simulink model "Integrated_LKS"  (Simulink 10.2)
settings: Solver=ode4  StartTime=0.0  StopTime=30  FixedStep=0.005  RelTol=1e-3  EnableMultiTasking=on
undefined symbols (not defined in the file or in its folder): sigbuilder_block
libraries: simulink x2
settings Model: Creator=Infineon02  LastModifiedBy=user
settings DataIOCC: SignalLoggingName=sigsOut
settings OptimizationCC: ExpressionDepthLimit=2147483647  InitFltsAndDblsToZero=on
settings DebuggingCC: SaveWithParameterizedLinksMsg=none  SignalResolutionControl=TryResolveAllWithWarning  MultiTaskDSMMsg=warning  MultiTaskCondExecSysMsg=none  StateNameClashWarn=warning
settings HardwareCC: TargetUnknown=on
settings GRTTargetCC: TargetFcnLib=ansi_tfl_tmw.mat

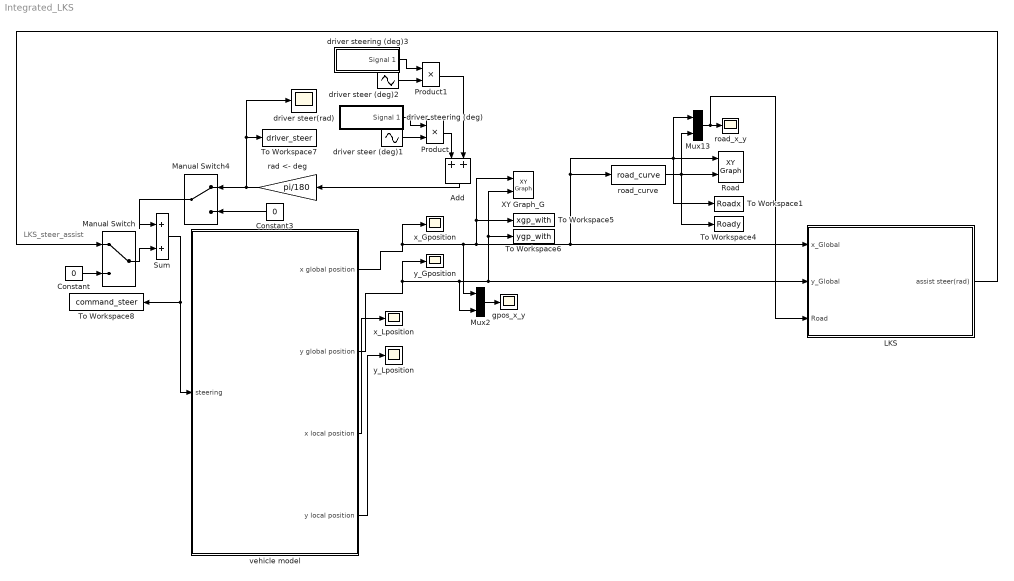
== system Integrated_LKS ==
  note: LKS_steer_assist
  Add : Sum
  Constant : Constant  Value=0
  Constant3 : Constant  Value=0
  LKS : Subsystem
  Manual Switch : ManualSwitch
  Manual Switch4 : ManualSwitch
  Mux13 : Mux  Inputs=2
  Mux2 : Mux  Inputs=2
  Product : Product  RndMeth=Zero
  Product1 : Product  RndMeth=Zero
  Road : simulink/Sinks/XY Graph  xmin=0  xmax=500  ymin=-100  ymax=1  st=0
  Sum : Sum  Inputs=|++  SaturateOnIntegerOverflow=on
  To Workspace1 : ToWorkspace  VariableName=Roadx  SampleTime=-1
  To Workspace4 : ToWorkspace  VariableName=Roady  SampleTime=-1
  To Workspace5 : ToWorkspace  VariableName=xgp_with  SampleTime=-1
  To Workspace6 : ToWorkspace  VariableName=ygp_with  SampleTime=-1
  To Workspace7 : ToWorkspace  VariableName=driver_steer  SampleTime=-1
  To Workspace8 : ToWorkspace  VariableName=command_steer  SampleTime=-1
  XY Graph_G : simulink/Sinks/XY Graph  xmin=0  xmax=500  ymin=-100  ymax=1  st=0
  driver steer (deg)1 : Sin  Amplitude=0.8  Frequency=0.34907  Phase=0.34898  SampleTime=0
  driver steer (deg)2 : Sin  Amplitude=0.8  Frequency=0.165347  Phase=2.64  SampleTime=0
  driver steer(rad) : Scope
  driver steering (deg) : Subsystem  Tag=STV Subsys  LoadFcn=sigbuilder_block('load');  StartFcn=sigbuilder_block('start');  StopFcn=sigbuilder_block('stop');  ClipboardFcn=sigbuilder_block('clipboard');  mask(Sigbuilder block){tuvar=[0:10]}
      mask help: Sigbuilder GUI
      mask init:
      | if ~strcmp(get_param(bdroot(gcbh),'SimulationStatus'),'stopped') tuvar = sigbuilder_block('maskInit'); end
      settings: CopyFcn=sigbuilder_block('copy');  DeleteFcn=sigbuilder_block('delete');  ModelCloseFcn=sigbuilder_block('modelClose');  PreSaveFcn=sigbuilder_block('preSave');  PauseFcn=sigbuilder_block('pause')  ContinueFcn=sigbuilder_block('continue')  NameChangeFcn=sigbuilder_block('namechange');  OpenFcn=sigbuilder_block('open',[-717 159.75 558.75 274.5 ]);  CloseFcn=sigbuilder_block('close');
      mask Display: plot(0, 0, 100, 100,[2, 2, 32, 32, 2], [68, 8, 8, 68, 68],[32, 2], [38, 38], [32, 19, 2],[53, 60, 44], [32, 17, 17, 2],[16, 16, 31, 31]);txt = getActiveGroup(gcbh);text(2, 100, txt,'verticalAlignment', 'top');
  driver steering (deg)3 : Subsystem  Tag=STV Subsys  LoadFcn=sigbuilder_block('load');  StartFcn=sigbuilder_block('start');  StopFcn=sigbuilder_block('stop');  ClipboardFcn=sigbuilder_block('clipboard');  mask(Sigbuilder block){tuvar=[0:10]}
      mask help: Sigbuilder GUI
      mask init:
      | if ~strcmp(get_param(bdroot(gcbh),'SimulationStatus'),'stopped') tuvar = sigbuilder_block('maskInit'); end
      settings: CopyFcn=sigbuilder_block('copy');  DeleteFcn=sigbuilder_block('delete');  ModelCloseFcn=sigbuilder_block('modelClose');  PreSaveFcn=sigbuilder_block('preSave');  PauseFcn=sigbuilder_block('pause')  ContinueFcn=sigbuilder_block('continue')  NameChangeFcn=sigbuilder_block('namechange');  OpenFcn=sigbuilder_block('open',[-723.75 76.5 558.75 274.5 ]);  CloseFcn=sigbuilder_block('close');
      mask Display: plot(0, 0, 100, 100,[2, 2, 32, 32, 2], [68, 8, 8, 68, 68],[32, 2], [38, 38], [32, 19, 2],[53, 60, 44], [32, 17, 17, 2],[16, 16, 31, 31]);txt = getActiveGroup(gcbh);text(2, 100, txt,'verticalAlignment', 'top');
  gpos_x_y : Scope
  rad <- deg : Gain  Gain=pi/180  SaturateOnIntegerOverflow=on  OutDataTypeStr=Inherit: Same as input  ParamDataTypeStr=Inherit: Same as input
  road_curve : MATLABFcn  MATLABFcn=road_curve
  road_x_y : Scope
  vehicle model : Subsystem
  x_Gposition : Scope
  x_Lposition : Scope
  y_Gposition : Scope
  y_Lposition : Scope
  wires:
  Constant/1 -> Manual Switch/2
  vehicle model/3(x local position) -> x_Lposition/1
  vehicle model/4(y local position) -> y_Lposition/1
  driver steer (deg)1/1 -> Product/2
  driver steering (deg)/1(Signal 1) -> Product/1
  Mux13/1 -> road_x_y/1, LKS/3(Road)
  road_curve/1 -> Mux13/2, Road/2, To Workspace4/1
  Manual Switch/1 -> Sum/2
  Sum/1 -> vehicle model/1(steering), To Workspace8/1
  vehicle model/1(x global position) -> x_Gposition/1, Mux13/1, Road/1, To Workspace1/1, road_curve/1, LKS/1(x_Global), To Workspace5/1, XY Graph_G/1, Mux2/1
  rad <- deg/1 -> Manual Switch4/1, driver steer(rad)/1, To Workspace7/1
  Manual Switch4/1 -> Sum/1
  Constant3/1 -> Manual Switch4/2
  vehicle model/2(y global position) -> y_Gposition/1, To Workspace6/1, XY Graph_G/2, LKS/2(y_Global), Mux2/2
  LKS/1(assist steer(rad)) -> Manual Switch/1
  Add/1 -> rad <- deg/1
  driver steer (deg)2/1 -> Product1/2
  driver steering (deg)3/1(Signal 1) -> Product1/1
  Product/1 -> Add/1
  Product1/1 -> Add/2
  Mux2/1 -> gpos_x_y/1

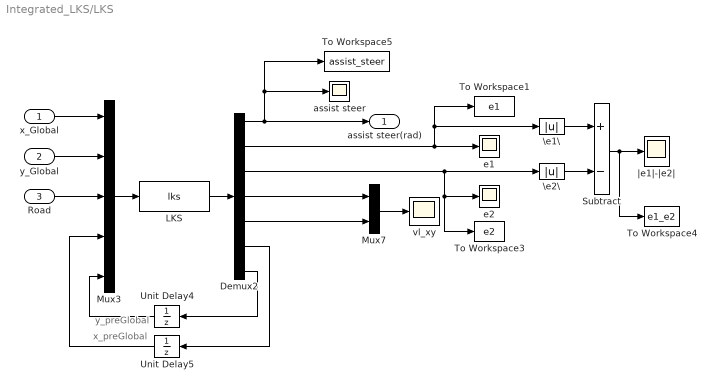
== system Integrated_LKS/LKS ==
  note: x_preGlobal
  note: y_preGlobal
  x_Global : Inport
  y_Global : Inport  Port=2
  Road : Inport  Port=3
  Demux2 : Demux  Outputs=7
  LKS : MATLABFcn  MATLABFcn=lks
  Mux3 : Mux  Inputs=5
  Mux7 : Mux  Inputs=2
  Subtract : Sum  Inputs=+-
  To Workspace1 : ToWorkspace  VariableName=e1  SampleTime=-1
  To Workspace3 : ToWorkspace  VariableName=e2  SampleTime=-1
  To Workspace4 : ToWorkspace  VariableName=e1_e2  SampleTime=-1
  To Workspace5 : ToWorkspace  VariableName=assist_steer  SampleTime=-1
  Unit Delay4 : UnitDelay  SampleTime=-1  HasFrameUpgradeWarning=on
  Unit Delay5 : UnitDelay  SampleTime=-1  HasFrameUpgradeWarning=on
  \e1\ : Abs
  \e2\ : Abs
  assist steer : Scope
  e1 : Scope
  e2 : Scope
  vl_xy : Scope
  |e1|-|e2| : Scope
  assist steer(rad) : Outport
  wires:
  Demux2/7 -> Unit Delay4/1
  Unit Delay4/1 -> Mux3/5
  Demux2/6 -> Unit Delay5/1
  Unit Delay5/1 -> Mux3/4
  Demux2/5 -> Mux7/2
  Demux2/4 -> Mux7/1
  Demux2/3 -> \e2\/1, e2/1, To Workspace3/1
  Mux7/1 -> vl_xy/1
  Demux2/2 -> e1/1, \e1\/1, To Workspace1/1
  Demux2/1 -> assist steer(rad)/1, assist steer/1, To Workspace5/1
  LKS/1 -> Demux2/1
  Mux3/1 -> LKS/1
  x_Global/1 -> Mux3/1
  y_Global/1 -> Mux3/2
  Road/1 -> Mux3/3
  \e1\/1 -> Subtract/1
  \e2\/1 -> Subtract/2
  Subtract/1 -> |e1|-|e2|/1, To Workspace4/1

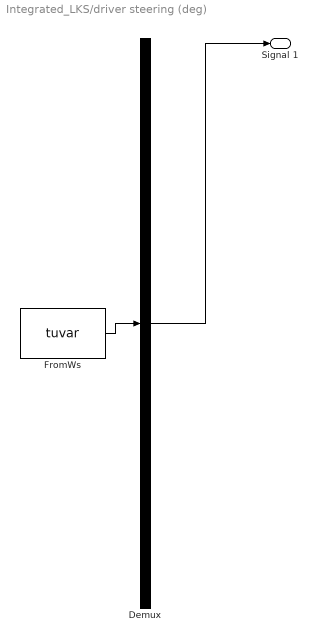
== system Integrated_LKS/driver steering (deg) ==
  Demux : Demux  Tag=STV Demux  Outputs=1
      settings: DisplayOption=none
  FromWs : FromWorkspace  Tag=STV FromWs  VariableName=tuvar  SigBuilderData=DataTag0  VnvData=DataTag1
      SigBuilderData=|
      | common.afterFinalStr = 'Extrapolate'
      | common.sampleTime = 0
      | dataSet.timeRange = [0 30]
      | dataSet.name = 'Group 1'
      | sbobj.Groups.Name = 'Group 1'
      | sbobj.Groups.Signals.Name = 'Signal 1'
      | sbobj.Groups.Signals.XData = [0 8 8 12.6 12.6 30]
      | sbobj.Groups.Signals.YData = [0 0 1 1 0 0]
      | sbobj.Groups.TimeRange = [0 30]
  Signal 1 : Outport  Tag=STV Outport
  wires:
  FromWs/1 -> Demux/1
  Demux/1 -> Signal 1/1

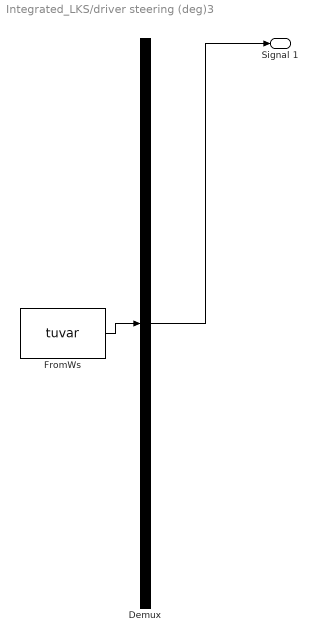
== system Integrated_LKS/driver steering (deg)3 ==
  Demux : Demux  Tag=STV Demux  Outputs=1
      settings: DisplayOption=none
  FromWs : FromWorkspace  Tag=STV FromWs  VariableName=tuvar  SigBuilderData=DataTag2  VnvData=DataTag3
      SigBuilderData=|
      | common.afterFinalStr = 'Extrapolate'
      | common.sampleTime = 0
      | dataSet.timeRange = [0 30]
      | dataSet.name = 'Group 1'
      | sbobj.Groups.Name = 'Group 1'
      | sbobj.Groups.Signals.Name = 'Signal 1'
      | sbobj.Groups.Signals.XData = [0 12.6 12.6 22 22 30]
      | sbobj.Groups.Signals.YData = [0 0 1 1 0 0]
      | sbobj.Groups.TimeRange = [0 30]
  Signal 1 : Outport  Tag=STV Outport
  wires:
  Demux/1 -> Signal 1/1
  FromWs/1 -> Demux/1

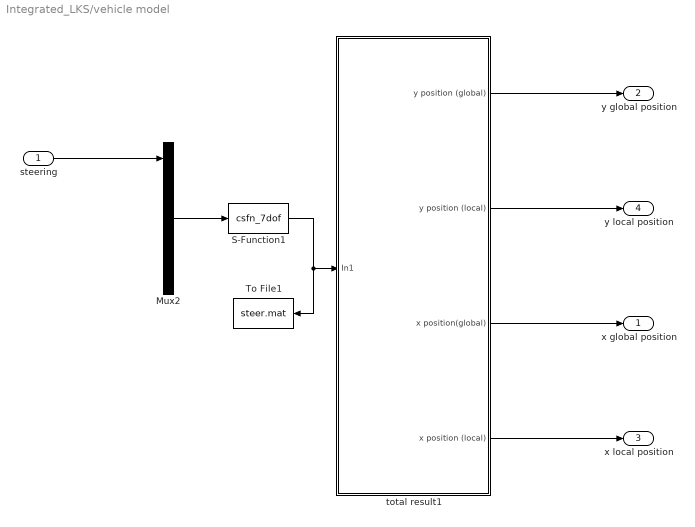
== system Integrated_LKS/vehicle model ==
  steering : Inport
  Mux2 : Mux  Inputs=5
  S-Function1 : S-Function  FunctionName=csfn_7dof  SFunctionDeploymentMode=off  EnableBusSupport=off
  To File1 : ToFile  Filename=steer.mat  MatrixName=steer
  total result1 : Subsystem
  x global position : Outport
  y global position : Outport  Port=2
  x local position : Outport  Port=3
  y local position : Outport  Port=4
  wires:
  S-Function1/1 -> total result1/1(In1), To File1/1
  steering/1 -> Mux2/1
  Mux2/1 -> S-Function1/1
  total result1/1(y position (global)) -> y global position/1
  total result1/2(y position (local)) -> y local position/1
  total result1/3(x position(global)) -> x global position/1
  total result1/4(x position (local)) -> x local position/1

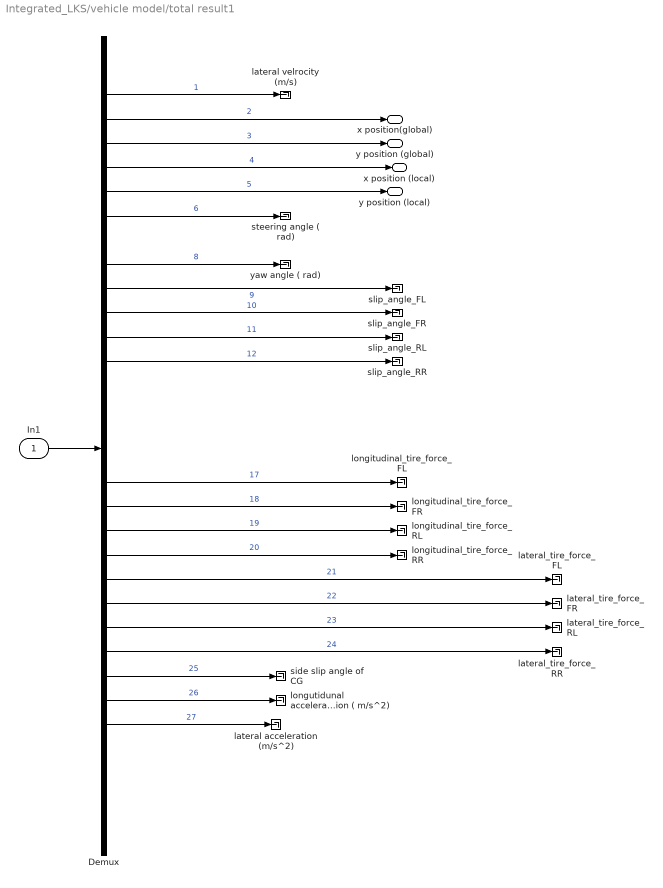
== system Integrated_LKS/vehicle model/total result1 ==
  In1 : Inport
  Demux : Demux  Outputs=32
      settings: DisplayOption=none
  lateral acceleration (m/s^2) : Terminator
  lateral velrocity (m/s) : Terminator
  lateral_tire_force_FL : Terminator
  lateral_tire_force_FR : Terminator
  lateral_tire_force_RL : Terminator
  lateral_tire_force_RR : Terminator
  longitudinal_tire_force_FL : Terminator
  longitudinal_tire_force_FR : Terminator
  longitudinal_tire_force_RL : Terminator
  longitudinal_tire_force_RR : Terminator
  longutidunal acceleration ( m/s^2) : Terminator
  side slip angle of CG : Terminator
  slip_angle_FL : Terminator
  slip_angle_FR : Terminator
  slip_angle_RL : Terminator
  slip_angle_RR : Terminator
  steering angle ( rad) : Terminator
  yaw angle ( rad) : Terminator
  y position (global) : Outport
  y position (local) : Outport  Port=2
  x position(global) : Outport  Port=3
  x position (local) : Outport  Port=4
  wires:
  Demux/2 -> lateral velrocity (m/s)/1  "1"
  Demux/3 -> x position(global)/1  "2"
  Demux/13 -> slip_angle_RR/1  "12"
  Demux/12 -> slip_angle_RL/1  "11"
  Demux/11 -> slip_angle_FR/1  "10"
  Demux/10 -> slip_angle_FL/1  "9"
  Demux/9 -> yaw angle ( rad)/1  "8"
  Demux/7 -> steering angle ( rad)/1  "6"
  Demux/6 -> y position (local)/1  "5"
  Demux/5 -> x position (local)/1  "4"
  Demux/4 -> y position (global)/1  "3"
  In1/1 -> Demux/1
  Demux/18 -> longitudinal_tire_force_FL/1  "17"
  Demux/19 -> longitudinal_tire_force_FR/1  "18"
  Demux/20 -> longitudinal_tire_force_RL/1  "19"
  Demux/21 -> longitudinal_tire_force_RR/1  "20"
  Demux/22 -> lateral_tire_force_FL/1  "21"
  Demux/23 -> lateral_tire_force_FR/1  "22"
  Demux/24 -> lateral_tire_force_RL/1  "23"
  Demux/25 -> lateral_tire_force_RR/1  "24"
  Demux/26 -> side slip angle of CG/1  "25"
  Demux/27 -> longutidunal acceleration ( m/s^2)/1  "26"
  Demux/28 -> lateral acceleration (m/s^2)/1  "27"
